simulink model "Simulacion"  (Simulink 7.5)
settings: Solver=ode45  StartTime=0.0  StopTime=10.0  RelTol=1e-3
settings Model: Creator=My Laptop  LastModifiedBy=My Laptop

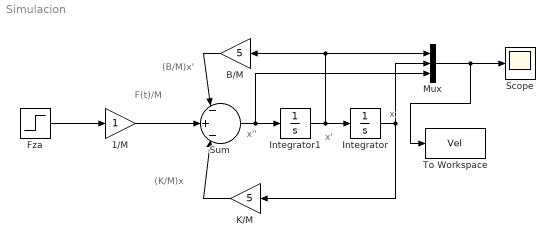
== system Simulacion ==
  note: x'
  note: x
  note: x''
  note: F(t)/M
  note: (B/M)x'
  note: (K/M)x
  1/M : Gain  ParameterDataType=fixdt(1, 16)  ParameterScaling=2^0  OutDataType=fixdt(1, 16)  OutScaling=2^0
  B/M : Gain  Gain=5  ParameterDataType=fixdt(1, 16)  ParameterScaling=2^0  OutDataType=fixdt(1, 16)  OutScaling=2^0
  Fza : Step  SampleTime=0
  Integrator : Integrator
  Integrator1 : Integrator
  K/M : Gain  Gain=5  ParameterDataType=fixdt(1, 16)  ParameterScaling=2^0  OutDataType=fixdt(1, 16)  OutScaling=2^0
  Mux : Mux  Inputs=3
  Scope : Scope
  Sum : Sum  Inputs=|-|+|-|  OutDataType=fixdt(1, 16)  OutScaling=2^0
  To Workspace : ToWorkspace  VariableName=Vel  SampleTime=-1  SaveFormat=Array
  wires:
  Fza/1 -> 1/M/1
  1/M/1 -> Sum/2
  B/M/1 -> Sum/1
  K/M/1 -> Sum/3
  Sum/1 -> Integrator1/1, Mux/3
  Integrator/1 -> K/M/1, Mux/2
  Integrator1/1 -> Integrator/1, B/M/1, Mux/1
  Mux/1 -> To Workspace/1, Scope/1
